simulink subsystem "subsystem_directDynamics"  (R2022a)
settings: Solver=VariableStepAuto  StartTime=0.0  StopTime=10.0  RelTol=1e-3
settings Model: Creator=Philipp  LastModifiedBy=Philipp
settings DebuggingCC: UnconnectedInputMsg=warning  UnconnectedOutputMsg=warning  UnconnectedLineMsg=warning
settings RTWCC: DLArmComputeVersion=19.05

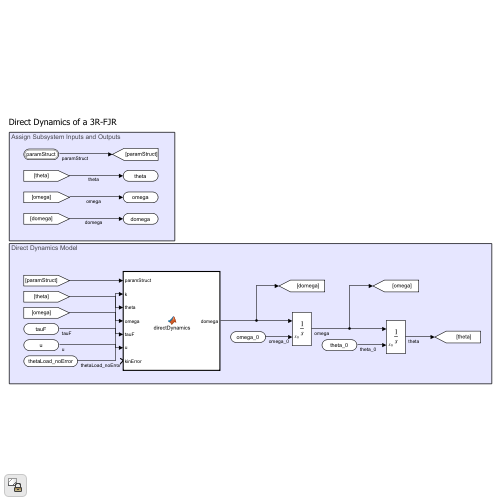
[thumbnail: Simulink's stored preview of the top-level diagram]
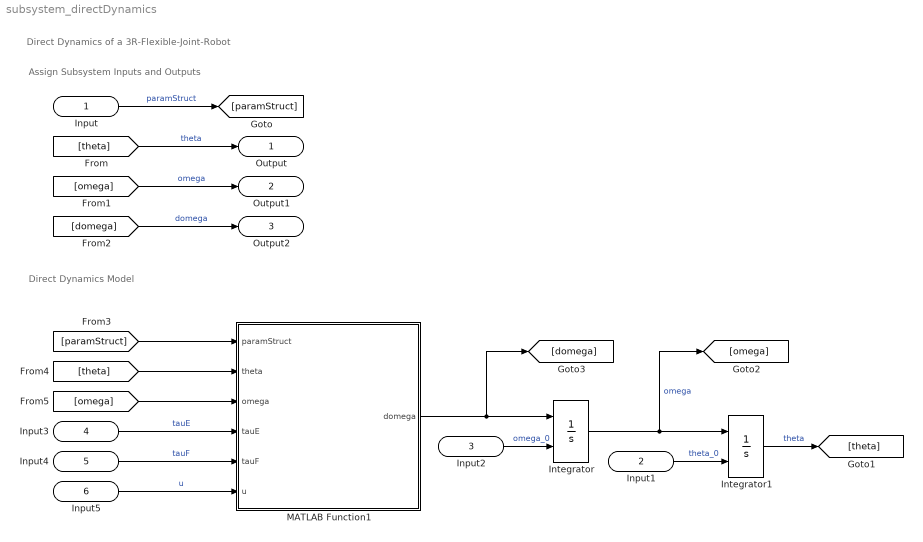
== system subsystem_directDynamics ==
  note: Direct Dynamics Model
  note: Assign Subsystem Inputs and Outputs
  note: Direct Dynamics of a 3R-Flexible-Joint-Robot
  Input : Inport  OutDataTypeStr=Bus: main_bus
  Input1 : Inport  Port=2
  Input2 : Inport  Port=3
  Input3 : Inport  Port=4
  Input4 : Inport  Port=5
  Input5 : Inport  Port=6
  Integrator : Integrator  InitialConditionSource=external
  Integrator1 : Integrator  InitialConditionSource=external
  MATLAB Function1 : MATLAB Function  TreatAsAtomicUnit=on
  Output : Outport  PortDimensions=6
  Output1 : Outport  Port=2  PortDimensions=6
  Output2 : Outport  Port=3  PortDimensions=6
  wires:
  Input5/1 -> MATLAB Function1/6(u)  "u"
  Input4/1 -> MATLAB Function1/5(tauF)  "tauF"
  Input3/1 -> MATLAB Function1/4(tauE)  "tauE"
  [omega] -> Output1/1  "omega"
  [domega] -> Output2/1  "domega"
  [theta] -> Output/1  "theta"
  Input/1 -> [paramStruct]  "paramStruct"
  [paramStruct] -> MATLAB Function1/1(paramStruct)
  [theta] -> MATLAB Function1/2(theta)
  [omega] -> MATLAB Function1/3(omega)
  MATLAB Function1/1(domega) -> Integrator/1, [domega]
  Input2/1 -> Integrator/2  "omega_0"
  Integrator/1 -> [omega], Integrator1/1  "omega"
  Input1/1 -> Integrator1/2  "theta_0"
  Integrator1/1 -> [theta]  "theta"

== matlab function subsystem_directDynamics/MATLAB Function1 ==
  data: paramStruct input; theta input; omega input; tauE input; domega output; tauF input; u input
function domega = directDynamics(paramStruct, theta, omega, tauE, tauF, u)

g = paramStruct.robot.g;
i_g = paramStruct.robot.i_g;
r_P1P2 = paramStruct.robot.r_P1P2;
r_P2P3 = paramStruct.robot.r_P2P3;
r_P3P4 = paramStruct.robot.r_P3P4;
baseParam = paramStruct.robot.baseParam;

if paramStruct.robot.comModel
    domega = directDynamics_complete_fun(g, i_g, r_P1P2, r_P2P3, r_P3P4, baseParam, theta, omega, tauE, tauF, u);
else
    domega = directDynamics_reduced_fun(g, i_g, r_P1P2, r_P2P3, r_P3P4, baseParam, theta, omega, tauE, tauF, u);
end
